simulink subsystem "TOAD_Controller_3"  (R2026a)
settings: Solver=VariableStepAuto
undefined symbols (not defined in the file or in its folder): constants6DoF, DiscIntNeverNeededParam, dt_SIM, u0
libraries: simulink x1
settings Model: Creator=pplat  LastModifiedBy=pplat

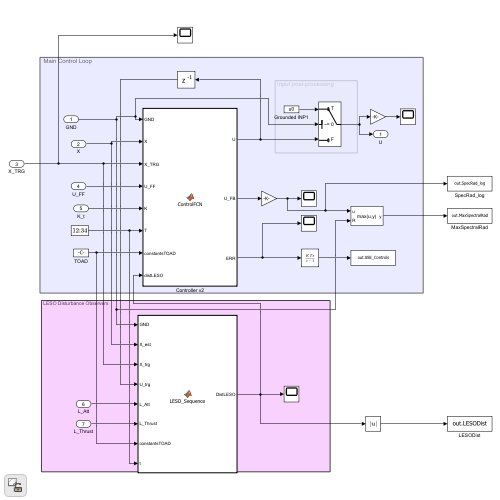
[thumbnail: Simulink's stored preview of the top-level diagram]
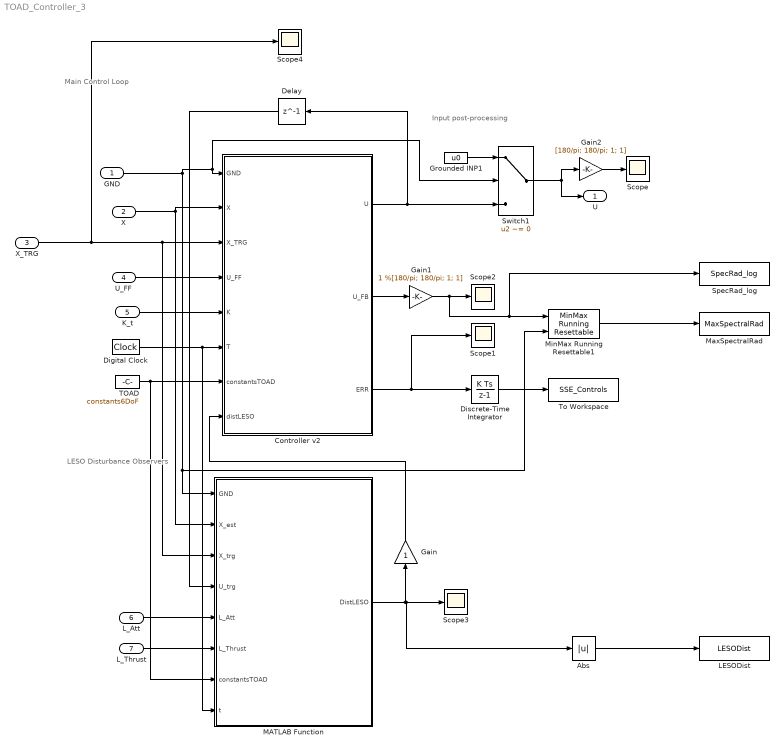
== system TOAD_Controller_3 ==
  note: LESO Disturbance Observers
  note: Main Control Loop
  note: Input post-processing
  GND : Inport
  X : Inport  Port=2
  X_TRG : Inport  Port=3
  U_FF : Inport  Port=4
  K_t : Inport  Port=5
  L_Att : Inport  Port=6
  L_Thrust : Inport  Port=7
  Abs : Abs  SaturateOnIntegerOverflow=off
  Controller v2 : MATLAB Function  TreatAsAtomicUnit=on
  Delay : Delay  DelayLength=1  InitialCondition=[0;0;constants6DoF.m_wet*constants6DoF.g;0]
  Digital Clock : DigitalClock  SampleTime=dt_SIM
  Discrete-Time Integrator : DiscreteIntegrator  InitialCondition=zeros(12,1)  SampleTime=-1  ICPrevOutput=DiscIntNeverNeededParam  ICPrevScaledInput=DiscIntNeverNeededParam
  Gain : Gain
  Gain1 : Gain  Gain=1 %[180/pi; 180/pi; 1; 1]
  Gain2 : Gain  Gain=[180/pi; 180/pi; 1; 1]
  Grounded INP1 : Constant  Value=u0
  LESODist : ToWorkspace  VariableName=LESODist  SaveFormat=Timeseries  SampleTime=0.1
  MATLAB Function : MATLAB Function  TreatAsAtomicUnit=on
  MaxSpectralRad : ToWorkspace  VariableName=MaxSpectralRad  SaveFormat=Timeseries  SampleTime=0.5
      settings: MaxDataPoints=1
  MinMax Running Resettable1 : simulink/Math Operations/MinMax Running Resettable  Function=max  vinit=0.0
  Scope{,1..4} (5 alike) : Scope
      Scope settings: ActiveDisplayYMinimum=-18.749999999999996  ActiveDisplayYMaximum=18.749999999999996  DataLoggingVariableName=ScopeData13
      Scope1 settings: ActiveDisplayYMinimum=-0.44115785504721572  ActiveDisplayYMaximum=0.93577139848826363  DataLoggingVariableName=ScopeData17
      Scope2 settings: ActiveDisplayYMinimum=0.98872199279041462  ActiveDisplayYMaximum=1.0015020648862691  DataLoggingVariableName=ScopeData18
      Scope3 settings: ActiveDisplayYMinimum=-5.9224528263127372  ActiveDisplayYMaximum=10.913487157856956  DataLoggingVariableName=ScopeData8
      Scope4 settings: ActiveDisplayYMinimum=-13.671494643450981  ActiveDisplayYMaximum=84.849943478640427  DataLoggingVariableName=ScopeData21
  SpecRad_log : ToWorkspace  VariableName=SpecRad_log  SaveFormat=Timeseries  SampleTime=0.05
  Switch1 : Switch  Criteria=u2 ~= 0  SaturateOnIntegerOverflow=off  InputSameDT=off
  TOAD : Constant  Value=constants6DoF  OutDataTypeStr=Bus: Vehicle_Bus
  To Workspace : ToWorkspace  VariableName=SSE_Controls  SampleTime=-1
      settings: MaxDataPoints=1
  U : Outport
  wires:
  Grounded INP1/1 -> Switch1/1
  Switch1/1 -> U/1, Gain2/1
  Discrete-Time Integrator/1 -> To Workspace/1
  Controller v2/1(U) -> Switch1/3, Delay/1
  Gain2/1 -> Scope/1
  Controller v2/3(ERR) -> Discrete-Time Integrator/1, Scope1/1
  X/1 -> MATLAB Function/2(X_est), Controller v2/2(X)
  X_TRG/1 -> MATLAB Function/3(X_trg), Controller v2/3(X_TRG), Scope4/1
  U_FF/1 -> Controller v2/4(U_FF)
  K_t/1 -> Controller v2/5(K)
  Digital Clock/1 -> MATLAB Function/8(t), Controller v2/6(T)
  TOAD/1 -> MATLAB Function/7(constantsTOAD), Controller v2/7(constantsTOAD)
  Controller v2/2(U_FB) -> Gain1/1
  Gain1/1 -> Scope2/1, MinMax Running Resettable1/1, SpecRad_log/1
  Delay/1 -> MATLAB Function/4(U_trg)
  L_Att/1 -> MATLAB Function/5(L_Att)
  L_Thrust/1 -> MATLAB Function/6(L_Thrust)
  MinMax Running Resettable1/1 -> MaxSpectralRad/1
  GND/1 -> MinMax Running Resettable1/2, MATLAB Function/1(GND), Switch1/2, Controller v2/1(GND)
  Abs/1 -> LESODist/1
  MATLAB Function/1(DistLESO) -> Gain/1, Scope3/1, Abs/1
  Gain/1 -> Controller v2/8(distLESO)

== matlab function TOAD_Controller_3/MATLAB Function ==
  data: GND input; X_est input; DistLESO output; X_trg input; U_trg input; L_Att input; L_Thrust input; constantsTOAD input; t input
function DistLESO = LESO_Sequence(GND, X_est, X_trg, U_trg, L_Att, L_Thrust, constantsTOAD, t)
    
    DistLESO = LESO_Sequence(GND, X_est, X_trg, U_trg, L_Att, L_Thrust, constantsTOAD, t);
end

== matlab function TOAD_Controller_3/Controller v2 ==
  data: GND input; X input; X_TRG input; U_FF input; K input; U output; U_FB output; T input; ERR output; constantsTOAD input; distLESO input
function [U, U_FB, ERR] = ControlFCN(GND, X, X_TRG, U_FF, K, T, constantsTOAD, distLESO)

    [U, U_FB, ERR] = TOAD_TVLQI_2(GND, X, X_TRG, U_FF, K, T, constantsTOAD, distLESO);
end
